simulink model "Date0501_QuadModel"  (R2015a)
settings: Solver=ode3  StartTime=0.0  StopTime=inf  FixedStep=Ts/5  RelTol=1e-3
values from neighbouring files (symbols this model uses):
  alpha1 = 10    [Date0501_Input_QuadModel.m]
  alpha2 = .3    (= 0.3)    [Date0501_Input_QuadModel.m]
  alpha3 = 1    [Date0501_Input_QuadModel.m]
  alpha4 = .1    (= 0.1)    [Date0501_Input_QuadModel.m]
  alpha5 = 1    [Date0501_Input_QuadModel.m]
  alpha6 = .1    (= 0.1)    [Date0501_Input_QuadModel.m]
  Am = - diag([10, 10, 10])*2    [Date0501_Input_QuadModel.m]
  Bm = diag([L_arm/Ix, L_arm/Iy, 1/Iz])    [Date0501_Input_QuadModel.m]
  Delay_Act = 0.0    (= 0)    [Date0501_Input_QuadModel.m]
  g = 9.81    [Date0501_Input_QuadModel.m]
  Inerita_Mat = diag([Ix, Iy, Iz])    [Date0501_Input_QuadModel.m]
  Ix = 7.5e-3    (= 0.0075)    [Date0501_Input_QuadModel.m]
  Iy = 7.5e-3    (= 0.0075)    [Date0501_Input_QuadModel.m]
  Jr = 6e-5    (= 6e-05)    [Date0501_Input_QuadModel.m]
  L_arm = 0.23    [Date0501_Input_QuadModel.m]
  m = 1.650    (= 1.65)    [Date0501_Input_QuadModel.m]
  Rotor_State_Fail = diag([1 1 1 0.5])    [Date0501_Input_QuadModel.m]
  Rotor_State_Normal = diag([1 1 1 1])    [Date0501_Input_QuadModel.m]
  Speed_Square_to_Thrust_N_Moment_Mat = [b b b b; 0 -b 0 b; -b 0 b 0; -d d -d d]    [Date0501_Input_QuadModel.m]
  Sum_Rotor_Angular_Velocity_Mat = [-1 1 -1 1]    [Date0501_Input_QuadModel.m]
  Ts = 0.005    [Date0501_Input_QuadModel.m]
libraries: simulink x8, cstblocks x4, etargetslib x1, aerolibutil x1, aerolibanimutils x1, dspnetwork x1
settings Model: SimulationMode=accelerator  Creator=hyoon33  LastModifiedBy=marinho
settings SolverCC: PositivePriorityOrder=on
settings DebuggingCC: UnderspecifiedInitializationDetection=Classic  MergeDetectMultiDrivingBlocksExec=none  SolverPrmCheckMsg=warning  StateNameClashWarn=warning

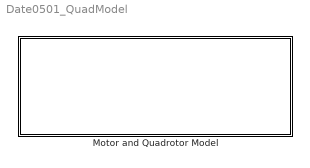
== system Date0501_QuadModel ==
  Motor and Quadrotor Model : Subsystem

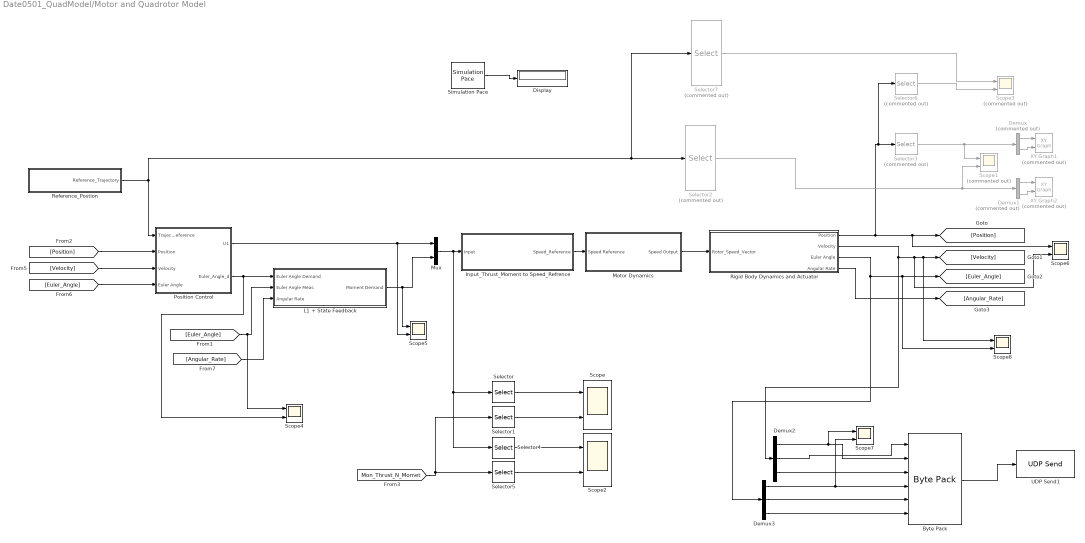
== system Date0501_QuadModel/Motor and Quadrotor Model ==
  Byte Pack : etargetslib/Byte Pack  datatypes={'double','double','double','double','double','double'}  byteAlign=1
  Demux : Demux  Commented=on  Outputs=2
  Demux1 : Demux  Commented=on  Outputs=2
  Demux2 : Demux  Outputs=3
  Demux3 : Demux  Outputs=3
  Display : Display
  Input_Thrust_Moment to Speed_Refrence : Subsystem
  L1 + State Feedback : Subsystem
  Motor Dynamics : Subsystem
  Mux : Mux  Inputs=2
  Position Control : Subsystem
  Reference_Postion : Subsystem
  Rigid Body Dynamics and Actuator : Subsystem
  Scope{,2,4..8} (7 alike) : Scope  NumInputPorts=2
      Scope settings: YMin=-0.6~-0.6  YMax=0.6~0.6
      Scope2 settings: YMin=6~6  YMax=13~13  SaveName=ScopeData11
      Scope4 settings: YMin=-0.175~-0.1  YMax=0.15~0.1  SaveName=ScopeData5
      Scope5 settings: YMin=-2.75~7.9  YMax=3~8.25  SaveName=ScopeData6
      Scope6 settings: YMin=-0.1~-0.7  YMax=1.3~0.6  SaveName=ScopeData7
      Scope7 settings: YMin=-1.5~-0.012  YMax=1.25~0.008  SaveName=ScopeData9
      Scope8 settings: YMin=-0.75~-0.075  YMax=1.25~0.125  SaveName=ScopeData10
  Scope1 : Scope  Commented=on  NumInputPorts=2
      settings: YMin=-0.8~-0.5  YMax=0.6~0.5  SaveName=ScopeData3
  Scope3 : Scope  Commented=on  NumInputPorts=2
      settings: YMin=1.02~0.91  YMax=1.095~0.985  SaveName=ScopeData12
  Selector : Selector  InputPortWidth=4  Indices=[2 3 4]
  Selector1 : Selector  InputPortWidth=4  Indices=[2 3 4]
  Selector2 : Selector  Commented=on  InputPortWidth=7  Indices=[3 5]
  Selector3 : Selector  Commented=on  InputPortWidth=3  Indices=[1 2]
  Selector4 : Selector  InputPortWidth=4  Indices=[1]
  Selector5 : Selector  InputPortWidth=4  Indices=[1]
  Selector6 : Selector  Commented=on  InputPortWidth=3  Indices=[3]
  Selector7 : Selector  Commented=on  InputPortWidth=7  Indices=[1]
  Simulation Pace : aerolibanimutils/Simulation Pace  SimulationPace=1  SleepMode=MATLAB Thread  OutputPaceError=on  SampleTime=-1
      settings: AttributesFormatString=%<SimulationPace> sec/sec
  UDP Send1 : dspnetwork/UDP Send  remoteURL='127.0.0.1'  remotePort=25000  localURL='0.0.0.0'  localPortSource=Automatically determine  localPort=-1  sampletime=-1  separateLengthPort=0
  XY Graph1 : simulink/Sinks/XY Graph  Commented=on  xmin=-2  xmax=2  ymin=-2  ymax=2  st=-1
  XY Graph2 : simulink/Sinks/XY Graph  Commented=on  xmin=-2  xmax=2  ymin=-2  ymax=2  st=-1
  wires:
  Rigid Body Dynamics and Actuator/4(Angular Rate) -> [Angular_Rate]
  Rigid Body Dynamics and Actuator/2(Velocity) -> Demux2/1, Scope6/2, Scope8/1, [Velocity]
  Rigid Body Dynamics and Actuator/1(Position) -> Selector6/1, Selector3/1, Scope6/1, [Position]
  Rigid Body Dynamics and Actuator/3(Euler Angle) -> Demux3/1, Scope8/2, [Euler_Angle]
  Input_Thrust_Moment to Speed_Refrence/1(Speed_Reference) -> Motor Dynamics/1(Speed Reference)
  L1 + State Feedback/1(Moment Demand) -> Scope5/1, Mux/2
  Reference_Postion/1(Reference_Trajectory) -> Position Control/1(Trajectory_Reference), Selector7/1, Selector2/1
  [Position] -> Position Control/2(Position)
  [Velocity] -> Position Control/3(Velocity)
  [Euler_Angle] -> Position Control/4(Euler Angle)
  [Euler_Angle] -> Scope4/1, L1 + State Feedback/2(Euler Angle Meas)
  [Angular_Rate] -> L1 + State Feedback/3(Angular Rate)
  Position Control/2(Euler_Angle_d) -> L1 + State Feedback/1(Euler Angle Demand), Scope4/2
  Mux/1 -> Selector/1, Selector4/1, Input_Thrust_Moment to Speed_Refrence/1(Input)
  Selector1/1 -> Scope/2
  Selector/1 -> Scope/1
  [Mon_Thrust_N_Momet] -> Selector5/1, Selector1/1
  Selector2/1 -> Scope1/2, Demux1/1
  Selector3/1 -> Scope1/1, Demux/1
  Selector4/1 -> Scope2/1
  Selector5/1 -> Scope2/2
  Selector6/1 -> Scope3/2
  Selector7/1 -> Scope3/1
  Position Control/1(U1) -> Mux/1, Scope5/2
  Demux1/1 -> XY Graph2/1
  Demux1/2 -> XY Graph2/2
  Demux/1 -> XY Graph1/1
  Demux/2 -> XY Graph1/2
  Byte Pack/1 -> UDP Send1/1
  Motor Dynamics/1(Speed Output) -> Rigid Body Dynamics and Actuator/1(Rotor_Speed_Vector)
  Simulation Pace/1 -> Display/1
  Demux2/1 -> Scope7/1, Byte Pack/2
  Demux3/2 -> Byte Pack/5
  Demux2/2 -> Byte Pack/1
  Demux3/1 -> Scope7/2, Byte Pack/4
  Demux2/3 -> Byte Pack/3
  Demux3/3 -> Byte Pack/6

== system Date0501_QuadModel/Motor and Quadrotor Model/Input_Thrust_Moment to Speed_Refrence ==
  Input : Inport
  From Speed 2 Thrust and Moment : Constant  Value=inv(Speed_Square_to_Thrust_N_Moment_Mat)  VectorParams1D=off
  Product : Product  Multiplication=Matrix(*)
  Speed_Reference : Outport
  wires:
  From Speed 2 Thrust and Moment/1 -> Product/1
  Product/1 -> Speed_Reference/1
  Input/1 -> Product/2

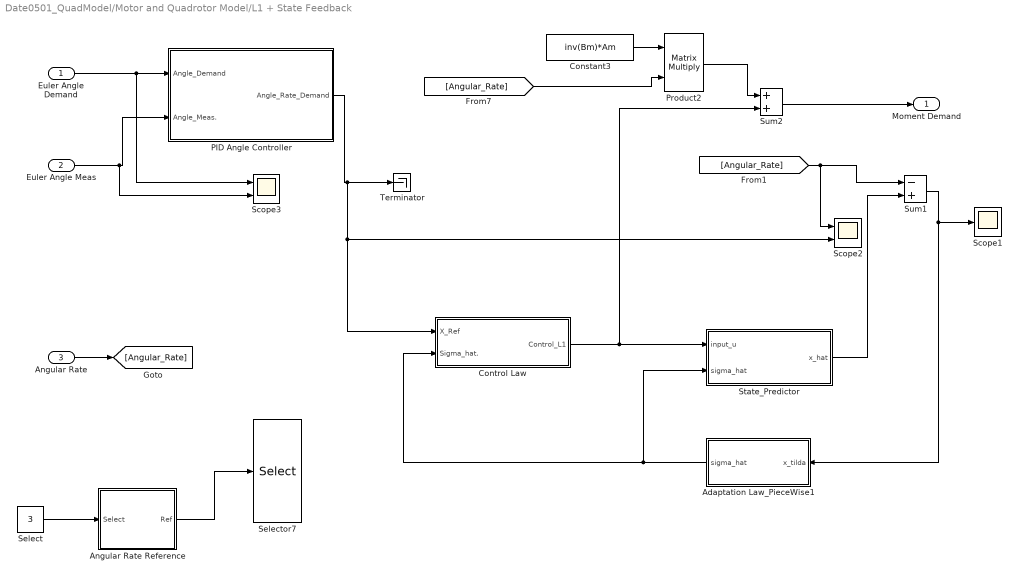
== system Date0501_QuadModel/Motor and Quadrotor Model/L1 + State Feedback ==
  Euler Angle Demand : Inport
  Euler Angle Meas : Inport  Port=2
  Angular Rate : Inport  Port=3
  Adaptation Law_PieceWise1 : Subsystem
  Angular Rate Reference : Subsystem
  Constant3 : Constant  Value=inv(Bm)*Am
  Control Law : Subsystem
  PID Angle Controller : Subsystem
  Product2 : Product  Multiplication=Matrix(*)
  Scope1 : Scope
      settings: YMin=-0.35  YMax=0.05  SaveName=ScopeData2
  Scope2 : Scope  NumInputPorts=2
      settings: YMin=-2~-3  YMax=2.5~3
  Scope3 : Scope  NumInputPorts=2
      settings: YMin=-1.75~-1.75  YMax=1.75~1.75  SaveName=ScopeData4
  Select : Constant  Value=3
  Selector7 : Selector  InputPortWidth=4  Indices=[1 2 3]
  State_Predictor : Subsystem
  Sum1 : Sum  Inputs=-+
  Sum2 : Sum
  Terminator : Terminator
  Moment Demand : Outport
  wires:
  Euler Angle Demand/1 -> Scope3/1, PID Angle Controller/1(Angle_Demand)
  Euler Angle Meas/1 -> Scope3/2, PID Angle Controller/2(Angle_Meas.)
  Angular Rate/1 -> [Angular_Rate]
  Sum1/1 -> Scope1/1, Adaptation Law_PieceWise1/1(x_tilda)
  State_Predictor/1(x_hat) -> Sum1/2
  Adaptation Law_PieceWise1/1(sigma_hat) -> State_Predictor/2(sigma_hat), Control Law/2(Sigma_hat.)
  PID Angle Controller/1(Angle_Rate_Demand) -> Scope2/2, Control Law/1(X_Ref), Terminator/1
  Constant3/1 -> Product2/1
  [Angular_Rate] -> Product2/2
  Sum2/1 -> Moment Demand/1
  Product2/1 -> Sum2/1
  Control Law/1(Control_L1) -> Sum2/2, State_Predictor/1(input_u)
  [Angular_Rate] -> Scope2/1, Sum1/1
  Select/1 -> Angular Rate Reference/1(Select)
  Angular Rate Reference/1(Ref) -> Selector7/1

== system Date0501_QuadModel/Motor and Quadrotor Model/Motor Dynamics ==
  Speed Reference : Inport
  Demux : Demux
  LTI System{1..4} (4 alike) : cstblocks/LTI System  sys=G_motor  IC=[]
  Mux : Mux
  Transport Delay : TransportDelay  DelayTime=Delay_Act
  Speed Output : Outport
  wires:
  Speed Reference/1 -> Transport Delay/1
  Transport Delay/1 -> Demux/1
  Mux/1 -> Speed Output/1
  Demux/1 -> LTI System1/1
  LTI System1/1 -> Mux/1
  Demux/2 -> LTI System2/1
  LTI System2/1 -> Mux/2
  Demux/3 -> LTI System3/1
  LTI System3/1 -> Mux/3
  Demux/4 -> LTI System4/1
  LTI System4/1 -> Mux/4

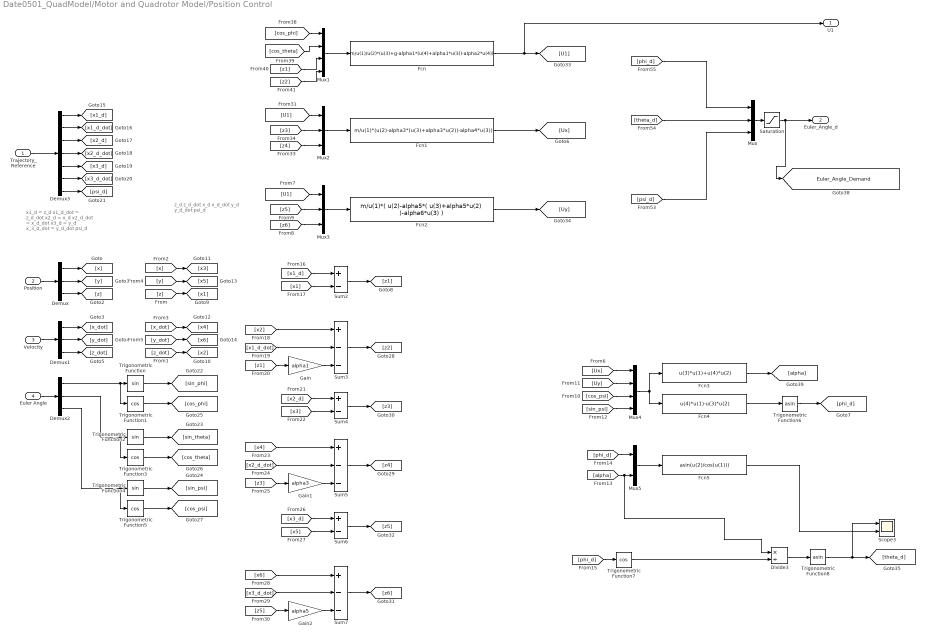
== system Date0501_QuadModel/Motor and Quadrotor Model/Position Control ==
  note: x1_d =  z_d
      | x1_d_dot = z_d_dot
      |
      | x2_d = x_d
      | x2_d_dot = x_d_dot
      |
      | x3_d = y_d
      | x_3_d_dot = y_d_dot
      |
      | psi_d
  note: z_d
      | z_d_dot
      |
      | x_d
      | x_d_dot
      |
      | y_d
      | y_d_dot
      |
      | psi_d
  Trajectory_Reference : Inport
  Position : Inport  Port=2
  Velocity : Inport  Port=3
  Euler Angle : Inport  Port=4
  Demux : Demux  Outputs=3
  Demux1 : Demux  Outputs=3
  Demux2 : Demux  Outputs=3
  Demux3 : Demux  Outputs=7
  Divide3 : Product  Inputs=*/
  Fcn : Fcn  Expr=m/u(1)/u(2)*(u(3)+g-alpha1*(u(4)+alpha1*u(3))-alpha2*u(4))
  Fcn1 : Fcn  Expr=m/u(1)*(u(2)-alpha3*(u(3)+alpha3*u(2))-alpha4*u(3))
  Fcn2 : Fcn  Expr=m/u(1)*( u(2)-alpha5*( u(3)+alpha5*u(2) )-alpha6*u(3) )
  Fcn3 : Fcn  Expr=u(3)*u(1)+u(4)*u(2)
  Fcn4 : Fcn  Expr=u(4)*u(1)-u(3)*u(2)
  Fcn5 : Fcn  Expr=asin(u(2)/cos(u(1)))
  Gain : Gain  Gain=alpha1
  Gain1 : Gain  Gain=alpha3
  Gain2 : Gain  Gain=alpha5
  Mux : Mux  Inputs=3
  Mux1 : Mux
  Mux2 : Mux  Inputs=3
  Mux3 : Mux  Inputs=3
  Mux4 : Mux
  Mux5 : Mux  Inputs=2
  Saturation : Saturate  UpperLimit=0.1  LowerLimit=-0.1
  Scope3 : Scope  NumInputPorts=2
      settings: YMin=-5~-5  YMax=5~5  SaveName=ScopeData8
  Sum2 : Sum  Inputs=+-
  Sum3 : Sum  Inputs=+--
  Sum4 : Sum  Inputs=+-
  Sum5 : Sum  Inputs=+--
  Sum6 : Sum  Inputs=+-
  Sum7 : Sum  Inputs=+--
  Trigonometric Function : Trigonometry
  Trigonometric Function{1,3,5,7} (4 alike) : Trigonometry  Operator=cos
  Trigonometric Function2 : Trigonometry
  Trigonometric Function4 : Trigonometry
  Trigonometric Function6 : Trigonometry  Operator=asin
  Trigonometric Function8 : Trigonometry  Operator=asin
  U1 : Outport
  Euler_Angle_d : Outport  Port=2
  tag scope: Euler_Angle_Demand=global
  wires:
  Position/1 -> Demux/1
  Velocity/1 -> Demux1/1
  Euler Angle/1 -> Demux2/1
  Demux/1 -> [x]
  Demux/2 -> [y]
  Demux/3 -> [z]
  Demux1/1 -> [x_dot]
  Demux1/2 -> [y_dot]
  Demux1/3 -> [z_dot]
  [z] -> [x1]
  [z_dot] -> [x2]
  [x] -> [x3]
  [x_dot] -> [x4]
  [y] -> [x5]
  [y_dot] -> [x6]
  Trajectory_Reference/1 -> Demux3/1
  Demux3/1 -> [x1_d]
  Demux3/2 -> [x1_d_dot]
  Demux3/3 -> [x2_d]
  Demux3/4 -> [x2_d_dot]
  Demux3/5 -> [x3_d]
  Demux3/6 -> [x3_d_dot]
  Demux3/7 -> [psi_d]
  Demux2/1 -> Trigonometric Function1/1, Trigonometric Function/1
  Trigonometric Function/1 -> [sin_phi]
  Trigonometric Function1/1 -> [cos_phi]
  Demux2/2 -> Trigonometric Function3/1, Trigonometric Function2/1
  Trigonometric Function2/1 -> [sin_theta]
  Trigonometric Function3/1 -> [cos_theta]
  Trigonometric Function4/1 -> [sin_psi]
  Trigonometric Function5/1 -> [cos_psi]
  Demux2/3 -> Trigonometric Function5/1, Trigonometric Function4/1
  [x1_d] -> Sum2/1
  [x1] -> Sum2/2
  Sum2/1 -> [z1]
  [x1_d_dot] -> Sum3/2
  [x2] -> Sum3/1
  Gain/1 -> Sum3/3
  [z1] -> Gain/1
  Sum3/1 -> [z2]
  [x2_d] -> Sum4/1
  [x3] -> Sum4/2
  Sum4/1 -> [z3]
  [x2_d_dot] -> Sum5/2
  [x4] -> Sum5/1
  Gain1/1 -> Sum5/3
  [z3] -> Gain1/1
  Sum5/1 -> [z4]
  [x3_d] -> Sum6/1
  [x5] -> Sum6/2
  Sum6/1 -> [z5]
  [x3_d_dot] -> Sum7/2
  [x6] -> Sum7/1
  Gain2/1 -> Sum7/3
  [z5] -> Gain2/1
  Sum7/1 -> [z6]
  Mux/1 -> Saturation/1
  [alpha] -> Divide3/1, Mux5/2
  Trigonometric Function7/1 -> Divide3/2
  Divide3/1 -> Trigonometric Function8/1
  Trigonometric Function8/1 -> Scope3/1, [theta_d]
  Mux1/1 -> Fcn/1
  [cos_phi] -> Mux1/1
  [cos_theta] -> Mux1/2
  [z1] -> Mux1/3
  [z2] -> Mux1/4
  Mux2/1 -> Fcn1/1
  [U1] -> Mux2/1
  [z4] -> Mux2/3
  [z3] -> Mux2/2
  Fcn1/1 -> [Ux]
  Mux3/1 -> Fcn2/1
  [U1] -> Mux3/1
  [z6] -> Mux3/3
  [z5] -> Mux3/2
  Fcn2/1 -> [Uy]
  Mux4/1 -> Fcn4/1, Fcn3/1
  [Ux] -> Mux4/1
  [cos_psi] -> Mux4/3
  [Uy] -> Mux4/2
  [sin_psi] -> Mux4/4
  Fcn4/1 -> Trigonometric Function6/1
  Trigonometric Function6/1 -> [phi_d]
  Fcn3/1 -> [alpha]
  [phi_d] -> Mux5/1
  Mux5/1 -> Fcn5/1
  Fcn5/1 -> Scope3/2
  [phi_d] -> Trigonometric Function7/1
  [phi_d] -> Mux/1
  [theta_d] -> Mux/2
  [psi_d] -> Mux/3
  Fcn/1 -> U1/1, [U1]
  Saturation/1 -> [Euler_Angle_Demand], Euler_Angle_d/1

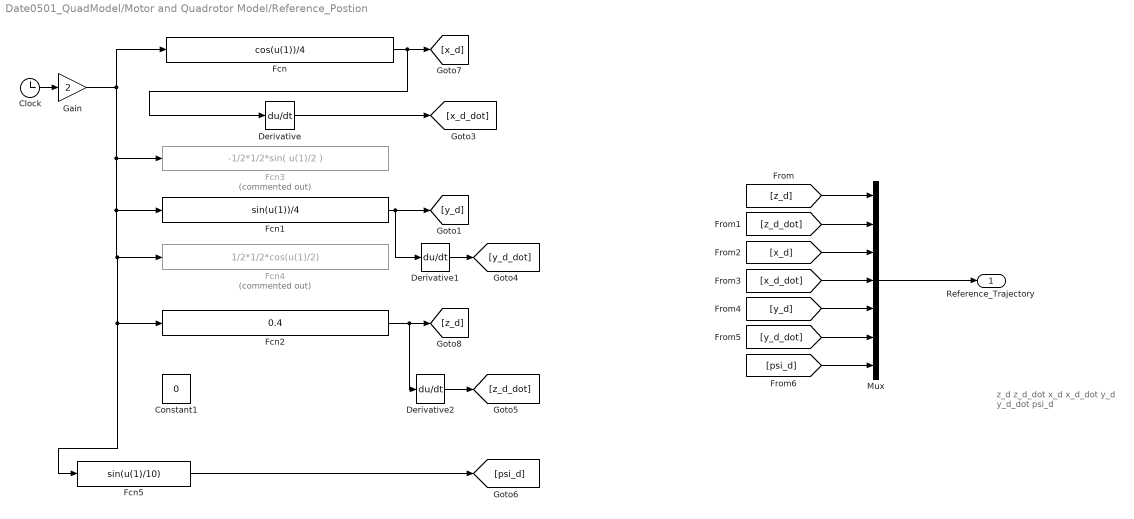
== system Date0501_QuadModel/Motor and Quadrotor Model/Reference_Postion ==
  note: z_d
      | z_d_dot
      |
      | x_d
      | x_d_dot
      |
      | y_d
      | y_d_dot
      |
      | psi_d
  Clock : Clock
  Constant1 : Constant  Value=0
  Derivative : Derivative
  Derivative1 : Derivative
  Derivative2 : Derivative
  Fcn : Fcn  Expr=cos(u(1))/4
  Fcn1 : Fcn  Expr=sin(u(1))/4
  Fcn2 : Fcn  Expr=0.4
  Fcn3 : Fcn  Commented=on  Expr=-1/2*1/2*sin( u(1)/2 )
  Fcn4 : Fcn  Commented=on  Expr=1/2*1/2*cos(u(1)/2)
  Fcn5 : Fcn  Expr=sin(u(1)/10)
  Gain : Gain  Gain=2
  Mux : Mux  Inputs=7
  Reference_Trajectory : Outport
  wires:
  Clock/1 -> Gain/1
  Fcn5/1 -> [psi_d]
  Mux/1 -> Reference_Trajectory/1
  [z_d] -> Mux/1
  [z_d_dot] -> Mux/2
  [x_d] -> Mux/3
  [x_d_dot] -> Mux/4
  [y_d] -> Mux/5
  [y_d_dot] -> Mux/6
  [psi_d] -> Mux/7
  Fcn2/1 -> Derivative2/1, [z_d]
  Gain/1 -> Fcn1/1, Fcn4/1, Fcn5/1, Fcn2/1, Fcn3/1, Fcn/1
  Fcn/1 -> [x_d], Derivative/1
  Derivative2/1 -> [z_d_dot]
  Fcn1/1 -> [y_d], Derivative1/1
  Derivative1/1 -> [y_d_dot]
  Derivative/1 -> [x_d_dot]

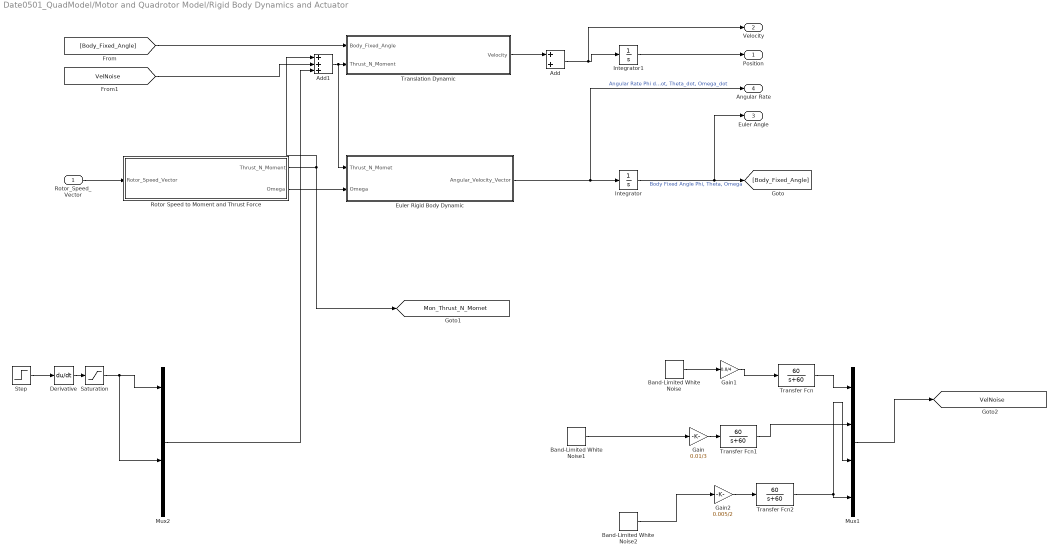
== system Date0501_QuadModel/Motor and Quadrotor Model/Rigid Body Dynamics and Actuator ==
  Rotor_Speed_Vector : Inport
  Add : Sum
  Add1 : Sum  Inputs=+++
  Band-Limited White Noise : simulink/Sources/Band-Limited White Noise  Cov=[.1]  Ts=Ts/5  seed=[23341]
  Band-Limited White Noise1 : simulink/Sources/Band-Limited White Noise  Cov=[.1]  Ts=Ts/5  seed=[24451]
  Band-Limited White Noise2 : simulink/Sources/Band-Limited White Noise  Cov=[.1]  Ts=Ts/5  seed=[87745]
  Derivative : Derivative
  Euler Rigid Body Dynamic : Subsystem
  Gain : Gain  Gain=0.01/3
  Gain1 : Gain  Gain=0.8/4
  Gain2 : Gain  Gain=0.005/2
  Integrator : Integrator
  Integrator1 : Integrator  InitialCondition=[0, 0, 0.5]'
  Mux1 : Mux
  Mux2 : Mux
  Rotor Speed to Moment and Thrust Force : Subsystem
  Saturation : Saturate  UpperLimit=10  LowerLimit=-10
  Step : Step  Time=20  SampleTime=0
  Transfer Fcn : TransferFcn  Numerator=[60]  Denominator=[1 60]
  Transfer Fcn1 : TransferFcn  Numerator=[60]  Denominator=[1 60]
  Transfer Fcn2 : TransferFcn  Numerator=[60]  Denominator=[1 60]
  Translation Dynamic : Subsystem
  Position : Outport
  Velocity : Outport  Port=2
  Euler Angle : Outport  Port=3
  Angular Rate : Outport  Port=4
  tag scope: Mon_Thrust_N_Momet=global, VelNoise=global
  wires:
  Rotor Speed to Moment and Thrust Force/1(Thrust_N_Moment) -> Add1/1, [Mon_Thrust_N_Momet]
  Euler Rigid Body Dynamic/1(Angular_Velocity_Vector) -> Integrator/1, Angular Rate/1  "Angular Rate Phi dot, Theta_dot, Omega_dot"
  Integrator/1 -> Euler Angle/1, [Body_Fixed_Angle]  "Body Fixed Angle Phi, Theta, Omega"
  Integrator1/1 -> Position/1
  Rotor Speed to Moment and Thrust Force/2(Omega) -> Euler Rigid Body Dynamic/2(Omega)
  Rotor_Speed_Vector/1 -> Rotor Speed to Moment and Thrust Force/1(Rotor_Speed_Vector)
  [Body_Fixed_Angle] -> Translation Dynamic/1(Body_Fixed_Angle)
  Band-Limited White Noise/1 -> Gain1/1
  Band-Limited White Noise1/1 -> Gain/1
  Band-Limited White Noise2/1 -> Gain2/1
  Mux1/1 -> [VelNoise]
  Gain/1 -> Transfer Fcn1/1
  Gain1/1 -> Transfer Fcn/1
  Gain2/1 -> Transfer Fcn2/1
  Translation Dynamic/1(Velocity) -> Add/1
  Add/1 -> Velocity/1, Integrator1/1
  Add1/1 -> Euler Rigid Body Dynamic/1(Thrust_N_Momet), Translation Dynamic/2(Thrust_N_Moment)
  Transfer Fcn/1 -> Mux1/1
  Transfer Fcn1/1 -> Mux1/2
  Transfer Fcn2/1 -> Mux1/3, Mux1/4
  [VelNoise] -> Add1/2
  Mux2/1 -> Add1/3
  Step/1 -> Derivative/1
  Derivative/1 -> Saturation/1
  Saturation/1 -> Mux2/3, Mux2/1

== system Date0501_QuadModel/Motor and Quadrotor Model/L1 + State Feedback/Adaptation Law_PieceWise1 ==
  x_tilda : Inport
  -inv(Bm)*inv(Phi_Ts)*exp_Am_Ts : Constant  Value=inv(Bm)*inv(inv(Am)*(expm(Am*Ts)-eye(3)))*(expm(Am*Ts))
  Gain3 : Gain  Gain=-1
  Product6 : Product  Multiplication=Matrix(*)
  Rate Transition : RateTransition  OutPortSampleTime=Ts
  Rate Transition1 : RateTransition  OutPortSampleTimeOpt=Inherit  OutPortSampleTime=Ts
  Rate Transition3 : RateTransition  X0=inv(Bm)*inv(inv(Am)*(exp(Am*Ts)-eye(3)))*(exp(Am*Ts))  OutPortSampleTime=Ts
  Saturation2 : Saturate  UpperLimit=10000  LowerLimit=-10000
  sigma_hat : Outport
  wires:
  Saturation2/1 -> sigma_hat/1
  Rate Transition3/1 -> Product6/1
  Gain3/1 -> Rate Transition1/1
  Rate Transition1/1 -> Saturation2/1
  -inv(Bm)*inv(Phi_Ts)*exp_Am_Ts/1 -> Rate Transition3/1
  x_tilda/1 -> Rate Transition/1
  Product6/1 -> Gain3/1
  Rate Transition/1 -> Product6/2

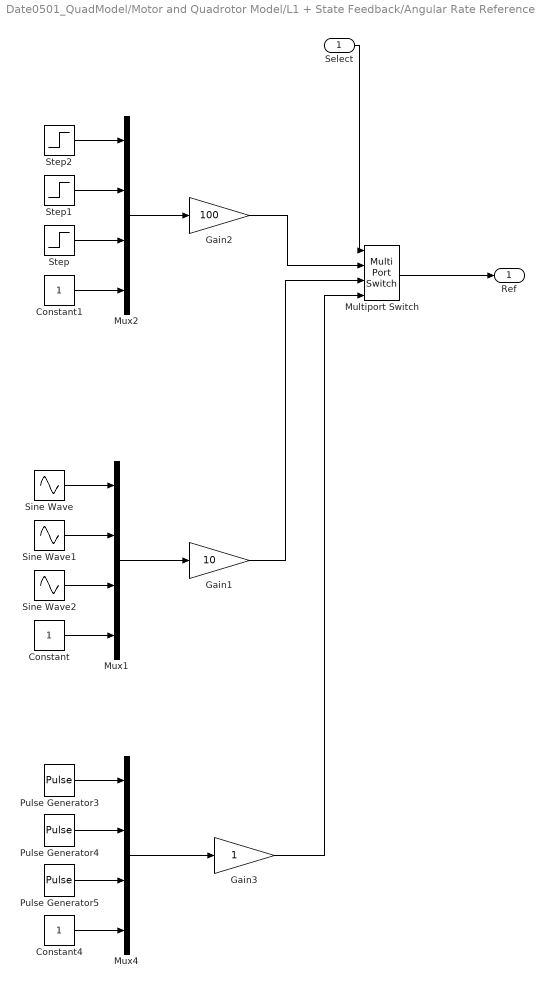
== system Date0501_QuadModel/Motor and Quadrotor Model/L1 + State Feedback/Angular Rate Reference ==
  Select : Inport
  Constant : Constant
  Constant1 : Constant
  Constant4 : Constant
  Gain1 : Gain  Gain=10
  Gain2 : Gain  Gain=100
  Gain3 : Gain
  Multiport Switch : MultiPortSwitch
  Mux1 : Mux
  Mux2 : Mux
  Mux4 : Mux
  Pulse Generator3 : DiscretePulseGenerator  PulseType=Time based  Period=8  PulseWidth=40  PhaseDelay=1
  Pulse Generator4 : DiscretePulseGenerator  PulseType=Time based  Period=8  PulseWidth=40  PhaseDelay=1.5
  Pulse Generator5 : DiscretePulseGenerator  PulseType=Time based  Amplitude=0  Period=8  PulseWidth=40  PhaseDelay=2
  Sine Wave : Sin  SampleTime=0
  Sine Wave1 : Sin  Phase=pi  SampleTime=0
  Sine Wave2 : Sin  Amplitude=0  SampleTime=0
  Step : Step  Time=3  After=0  SampleTime=0
  Step1 : Step  Time=2  SampleTime=0
  Step2 : Step  SampleTime=0
  Ref : Outport
  wires:
  Sine Wave/1 -> Mux1/1
  Sine Wave1/1 -> Mux1/2
  Sine Wave2/1 -> Mux1/3
  Constant/1 -> Mux1/4
  Step2/1 -> Mux2/1
  Step1/1 -> Mux2/2
  Step/1 -> Mux2/3
  Constant1/1 -> Mux2/4
  Mux1/1 -> Gain1/1
  Mux2/1 -> Gain2/1
  Select/1 -> Multiport Switch/1
  Gain2/1 -> Multiport Switch/2
  Multiport Switch/1 -> Ref/1
  Pulse Generator3/1 -> Mux4/1
  Pulse Generator4/1 -> Mux4/2
  Pulse Generator5/1 -> Mux4/3
  Constant4/1 -> Mux4/4
  Mux4/1 -> Gain3/1
  Gain1/1 -> Multiport Switch/3
  Gain3/1 -> Multiport Switch/4

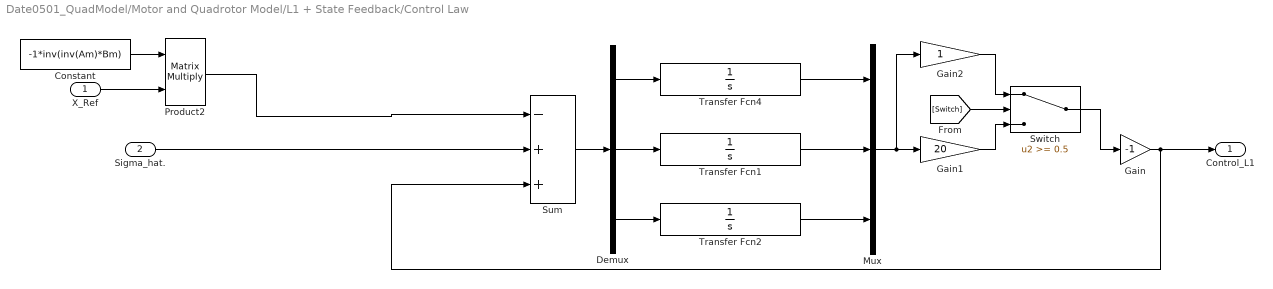
== system Date0501_QuadModel/Motor and Quadrotor Model/L1 + State Feedback/Control Law ==
  X_Ref : Inport
  Sigma_hat. : Inport  Port=2
  Constant : Constant  Value=-1*inv(inv(Am)*Bm)
  Demux : Demux  Outputs=3
  Gain : Gain  Gain=-1
  Gain1 : Gain  Gain=20
  Gain2 : Gain
  Mux : Mux  Inputs=3
  Product2 : Product  Multiplication=Matrix(*)
  Sum : Sum  Inputs=-++
  Switch : Switch  Threshold=0.5
  Transfer Fcn1 : TransferFcn  Denominator=[1 0]
  Transfer Fcn2 : TransferFcn  Denominator=[1 0]
  Transfer Fcn4 : TransferFcn  Denominator=[1 0]
  Control_L1 : Outport
  wires:
  X_Ref/1 -> Product2/2
  Sum/1 -> Demux/1
  Demux/1 -> Transfer Fcn4/1
  Demux/2 -> Transfer Fcn1/1
  Demux/3 -> Transfer Fcn2/1
  Mux/1 -> Gain2/1, Gain1/1
  Transfer Fcn4/1 -> Mux/1
  Transfer Fcn1/1 -> Mux/2
  Transfer Fcn2/1 -> Mux/3
  Constant/1 -> Product2/1
  Gain1/1 -> Switch/3
  Sigma_hat./1 -> Sum/2
  Gain/1 -> Sum/3, Control_L1/1
  Product2/1 -> Sum/1
  Gain2/1 -> Switch/1
  Switch/1 -> Gain/1
  [Switch] -> Switch/2

== system Date0501_QuadModel/Motor and Quadrotor Model/L1 + State Feedback/PID Angle Controller ==
  Angle_Demand : Inport
  Angle_Meas. : Inport  Port=2
  Demux : Demux  Outputs=3
  Demux1 : Demux  Outputs=3
  Mux : Mux  Inputs=3
  PID Controller (2DOF) : simulink/Continuous/PID Controller (2DOF)  Controller=PID  TimeDomain=Continuous-time  SampleTime=-1  IntegratorMethod=Forward Euler  FilterMethod=Forward Euler  Form=Parallel  UseFilter=on  ControllerParametersSource=internal  P=10  I=0.1  D=0.01  N=100  b=1  c=1  InitialConditionSource=internal  InitialConditionForIntegrator=0  InitialConditionForFilter=0  ExternalReset=none  LimitOutput=off  UpperSaturationLimit=inf  LowerSaturationLimit=-inf  LinearizeAsGain=on  AntiWindupMode=none  Kb=1  TrackingMode=off  Kt=1  PParamMin=[]  PParamMax=[]  IParamMin=[]  IParamMax=[]  DParamMin=[]  DParamMax=[]  NParamMin=[]  NParamMax=[]  bParamMin=[]  bParamMax=[]  cParamMin=[]  cParamMax=[]  KbParamMin=[]  KbParamMax=[]  KtParamMin=[]  KtParamMax=[]  POutMin=[]  POutMax=[]  IOutMin=[]  IOutMax=[]  DOutMin=[]  DOutMax=[]  NOutMin=[]  NOutMax=[]  bOutMin=[]  bOutMax=[]  cOutMin=[]  cOutMax=[]  KbOutMin=[]  KbOutMax=[]  KtOutMin=[]  KtOutMax=[]  IntegratorOutMin=[]  IntegratorOutMax=[]  FilterOutMin=[]  FilterOutMax=[]  SumOutMin=[]  SumOutMax=[]  Sum1OutMin=[]  Sum1OutMax=[]  Sum2OutMin=[]  Sum2OutMax=[]  Sum3OutMin=[]  Sum3OutMax=[]  SumI1OutMin=[]  SumI1OutMax=[]  SumI2OutMin=[]  SumI2OutMax=[]  SumI3OutMin=[]  SumI3OutMax=[]  SumDOutMin=[]  SumDOutMax=[]  SaturationOutMin=[]  SaturationOutMax=[]  IntegratorContinuousStateAttributes=''  IntegratorStateMustResolveToSignalObject=off  IntegratorRTWStateStorageClass=Auto  FilterContinuousStateAttributes=''  FilterStateMustResolveToSignalObject=off  FilterRTWStateStorageClass=Auto  DifferentiatorICPrevScaledInput=0  DifferentiatorOutMin=[]  DifferentiatorOutMax=[]
  PID Controller (2DOF)1 : simulink/Continuous/PID Controller (2DOF)  Controller=PID  TimeDomain=Continuous-time  SampleTime=-1  IntegratorMethod=Forward Euler  FilterMethod=Forward Euler  Form=Parallel  UseFilter=on  ControllerParametersSource=internal  P=10  I=0.1  D=0.01  N=100  b=1  c=1  InitialConditionSource=internal  InitialConditionForIntegrator=0  InitialConditionForFilter=0  ExternalReset=none  LimitOutput=off  UpperSaturationLimit=inf  LowerSaturationLimit=-inf  LinearizeAsGain=on  AntiWindupMode=none  Kb=1  TrackingMode=off  Kt=1  PParamMin=[]  PParamMax=[]  IParamMin=[]  IParamMax=[]  DParamMin=[]  DParamMax=[]  NParamMin=[]  NParamMax=[]  bParamMin=[]  bParamMax=[]  cParamMin=[]  cParamMax=[]  KbParamMin=[]  KbParamMax=[]  KtParamMin=[]  KtParamMax=[]  POutMin=[]  POutMax=[]  IOutMin=[]  IOutMax=[]  DOutMin=[]  DOutMax=[]  NOutMin=[]  NOutMax=[]  bOutMin=[]  bOutMax=[]  cOutMin=[]  cOutMax=[]  KbOutMin=[]  KbOutMax=[]  KtOutMin=[]  KtOutMax=[]  IntegratorOutMin=[]  IntegratorOutMax=[]  FilterOutMin=[]  FilterOutMax=[]  SumOutMin=[]  SumOutMax=[]  Sum1OutMin=[]  Sum1OutMax=[]  Sum2OutMin=[]  Sum2OutMax=[]  Sum3OutMin=[]  Sum3OutMax=[]  SumI1OutMin=[]  SumI1OutMax=[]  SumI2OutMin=[]  SumI2OutMax=[]  SumI3OutMin=[]  SumI3OutMax=[]  SumDOutMin=[]  SumDOutMax=[]  SaturationOutMin=[]  SaturationOutMax=[]  IntegratorContinuousStateAttributes=''  IntegratorStateMustResolveToSignalObject=off  IntegratorRTWStateStorageClass=Auto  FilterContinuousStateAttributes=''  FilterStateMustResolveToSignalObject=off  FilterRTWStateStorageClass=Auto  DifferentiatorICPrevScaledInput=0  DifferentiatorOutMin=[]  DifferentiatorOutMax=[]
  PID Controller (2DOF)2 : simulink/Continuous/PID Controller (2DOF)  Controller=PID  TimeDomain=Continuous-time  SampleTime=-1  IntegratorMethod=Forward Euler  FilterMethod=Forward Euler  Form=Parallel  UseFilter=on  ControllerParametersSource=internal  P=1  I=0.1  D=0.01  N=100  b=1  c=1  InitialConditionSource=internal  InitialConditionForIntegrator=0  InitialConditionForFilter=0  ExternalReset=none  LimitOutput=off  UpperSaturationLimit=inf  LowerSaturationLimit=-inf  LinearizeAsGain=on  AntiWindupMode=none  Kb=1  TrackingMode=off  Kt=1  PParamMin=[]  PParamMax=[]  IParamMin=[]  IParamMax=[]  DParamMin=[]  DParamMax=[]  NParamMin=[]  NParamMax=[]  bParamMin=[]  bParamMax=[]  cParamMin=[]  cParamMax=[]  KbParamMin=[]  KbParamMax=[]  KtParamMin=[]  KtParamMax=[]  POutMin=[]  POutMax=[]  IOutMin=[]  IOutMax=[]  DOutMin=[]  DOutMax=[]  NOutMin=[]  NOutMax=[]  bOutMin=[]  bOutMax=[]  cOutMin=[]  cOutMax=[]  KbOutMin=[]  KbOutMax=[]  KtOutMin=[]  KtOutMax=[]  IntegratorOutMin=[]  IntegratorOutMax=[]  FilterOutMin=[]  FilterOutMax=[]  SumOutMin=[]  SumOutMax=[]  Sum1OutMin=[]  Sum1OutMax=[]  Sum2OutMin=[]  Sum2OutMax=[]  Sum3OutMin=[]  Sum3OutMax=[]  SumI1OutMin=[]  SumI1OutMax=[]  SumI2OutMin=[]  SumI2OutMax=[]  SumI3OutMin=[]  SumI3OutMax=[]  SumDOutMin=[]  SumDOutMax=[]  SaturationOutMin=[]  SaturationOutMax=[]  IntegratorContinuousStateAttributes=''  IntegratorStateMustResolveToSignalObject=off  IntegratorRTWStateStorageClass=Auto  FilterContinuousStateAttributes=''  FilterStateMustResolveToSignalObject=off  FilterRTWStateStorageClass=Auto  DifferentiatorICPrevScaledInput=0  DifferentiatorOutMin=[]  DifferentiatorOutMax=[]
  Angle_Rate_Demand : Outport
  wires:
  Demux1/2 -> PID Controller (2DOF)1/2
  Demux/2 -> PID Controller (2DOF)1/1
  Angle_Meas./1 -> Demux1/1
  Demux1/1 -> PID Controller (2DOF)/2
  Demux/1 -> PID Controller (2DOF)/1
  Demux1/3 -> PID Controller (2DOF)2/2
  Angle_Demand/1 -> Demux/1
  Demux/3 -> PID Controller (2DOF)2/1
  PID Controller (2DOF)/1 -> Mux/1
  PID Controller (2DOF)1/1 -> Mux/2
  PID Controller (2DOF)2/1 -> Mux/3
  Mux/1 -> Angle_Rate_Demand/1

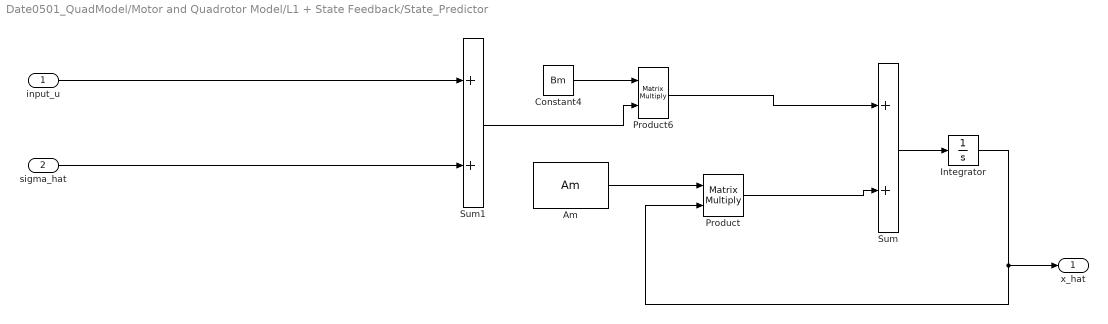
== system Date0501_QuadModel/Motor and Quadrotor Model/L1 + State Feedback/State_Predictor ==
  input_u : Inport
  sigma_hat : Inport  Port=2
  Am : Constant  Value=Am
  Constant4 : Constant  Value=Bm
  Integrator : Integrator
  Product : Product  Multiplication=Matrix(*)  RndMeth=Zero
  Product6 : Product  Multiplication=Matrix(*)
  Sum : Sum
  Sum1 : Sum
  x_hat : Outport
  wires:
  Product6/1 -> Sum/1
  Product/1 -> Sum/2
  Sum1/1 -> Product6/2
  Constant4/1 -> Product6/1
  Sum/1 -> Integrator/1
  input_u/1 -> Sum1/1
  Am/1 -> Product/1
  Integrator/1 -> x_hat/1, Product/2
  sigma_hat/1 -> Sum1/2

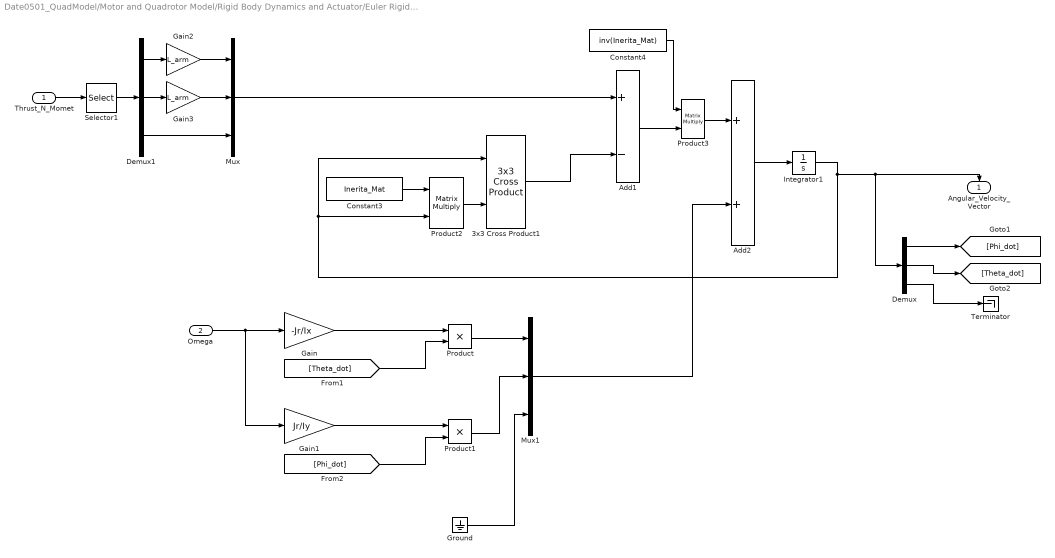
== system Date0501_QuadModel/Motor and Quadrotor Model/Rigid Body Dynamics and Actuator/Euler Rigid Body Dynamic ==
  Thrust_N_Momet : Inport
  Omega : Inport  Port=2
  3x3 Cross Product1 : aerolibutil/3x3 Cross Product
  Add1 : Sum  Inputs=+-
  Add2 : Sum
  Constant3 : Constant  Value=Inerita_Mat
  Constant4 : Constant  Value=inv(Inerita_Mat)
  Demux : Demux  Outputs=3
  Demux1 : Demux  Outputs=3
  Gain : Gain  Gain=-Jr/Ix
  Gain1 : Gain  Gain=Jr/Iy
  Gain2 : Gain  Gain=L_arm
  Gain3 : Gain  Gain=L_arm
  Ground : Ground
  Integrator1 : Integrator  InitialCondition=[0 0 0]
  Mux : Mux  Inputs=3
  Mux1 : Mux  Inputs=3
  Product : Product
  Product1 : Product
  Product2 : Product  Multiplication=Matrix(*)
  Product3 : Product  Multiplication=Matrix(*)
  Selector1 : Selector  InputPortWidth=4  Indices=[2 3 4]
  Terminator : Terminator
  Angular_Velocity_Vector : Outport
  wires:
  Add1/1 -> Product3/2
  3x3 Cross Product1/1 -> Add1/2
  Constant3/1 -> Product2/1
  Product2/1 -> 3x3 Cross Product1/2
  Constant4/1 -> Product3/1
  Thrust_N_Momet/1 -> Selector1/1
  Integrator1/1 -> Angular_Velocity_Vector/1, Demux/1, 3x3 Cross Product1/1, Product2/2
  Demux/1 -> [Phi_dot]
  Demux/2 -> [Theta_dot]
  Demux/3 -> Terminator/1
  Gain/1 -> Product/1
  Omega/1 -> Gain1/1, Gain/1
  [Theta_dot] -> Product/2
  Gain1/1 -> Product1/1
  [Phi_dot] -> Product1/2
  Selector1/1 -> Demux1/1
  Gain2/1 -> Mux/1
  Demux1/1 -> Gain2/1
  Demux1/2 -> Gain3/1
  Gain3/1 -> Mux/2
  Demux1/3 -> Mux/3
  Mux/1 -> Add1/1
  Product/1 -> Mux1/1
  Product1/1 -> Mux1/2
  Ground/1 -> Mux1/3
  Product3/1 -> Add2/1
  Add2/1 -> Integrator1/1
  Mux1/1 -> Add2/2

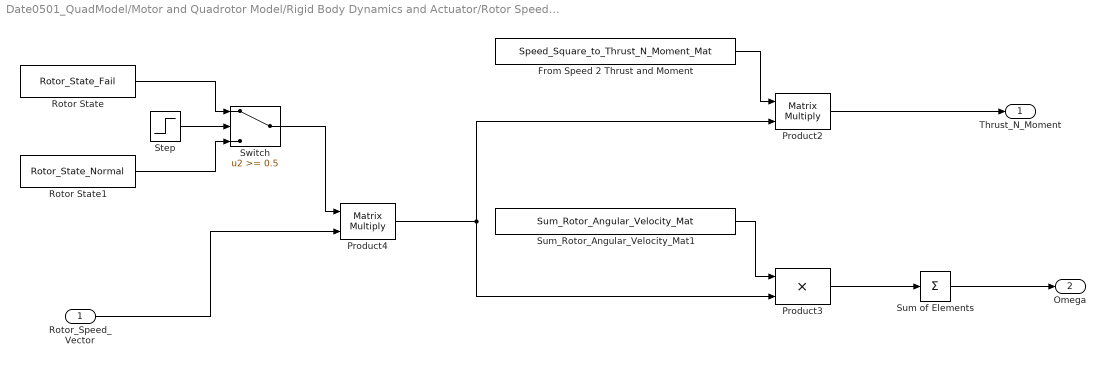
== system Date0501_QuadModel/Motor and Quadrotor Model/Rigid Body Dynamics and Actuator/Rotor Speed to Moment and Thrust Force ==
  Rotor_Speed_Vector : Inport
  From Speed 2 Thrust and Moment : Constant  Value=Speed_Square_to_Thrust_N_Moment_Mat
  Product2 : Product  Multiplication=Matrix(*)
  Product3 : Product
  Product4 : Product  Multiplication=Matrix(*)
  Rotor State : Constant  Value=Rotor_State_Fail
  Rotor State1 : Constant  Value=Rotor_State_Normal
  Step : Step  Time=10  SampleTime=0
  Sum of Elements : Sum  Inputs=+
  Sum_Rotor_Angular_Velocity_Mat1 : Constant  Value=Sum_Rotor_Angular_Velocity_Mat
  Switch : Switch  Threshold=0.5
  Thrust_N_Moment : Outport
  Omega : Outport  Port=2
  wires:
  From Speed 2 Thrust and Moment/1 -> Product2/1
  Rotor State/1 -> Switch/1
  Product4/1 -> Product2/2, Product3/2
  Switch/1 -> Product4/1
  Rotor State1/1 -> Switch/3
  Step/1 -> Switch/2
  Rotor_Speed_Vector/1 -> Product4/2
  Product2/1 -> Thrust_N_Moment/1
  Sum_Rotor_Angular_Velocity_Mat1/1 -> Product3/1
  Product3/1 -> Sum of Elements/1
  Sum of Elements/1 -> Omega/1

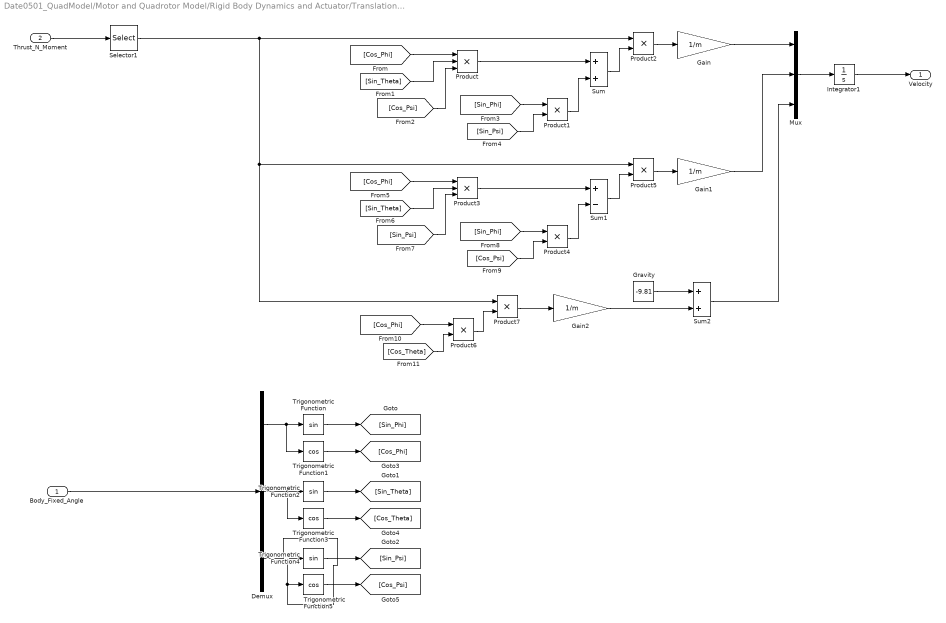
== system Date0501_QuadModel/Motor and Quadrotor Model/Rigid Body Dynamics and Actuator/Translation Dynamic ==
  Body_Fixed_Angle : Inport
  Thrust_N_Moment : Inport  Port=2
  Demux : Demux  Outputs=3
  Gain : Gain  Gain=1/m
  Gain1 : Gain  Gain=1/m
  Gain2 : Gain  Gain=1/m
  Gravity : Constant  Value=-9.81
  Integrator1 : Integrator  InitialCondition=[0 0 0]
  Mux : Mux  Inputs=3
  Product : Product  Inputs=3
  Product{1..2,4..7} (6 alike) : Product
  Product3 : Product  Inputs=3
  Selector1 : Selector  InputPortWidth=4  Indices=[1]
  Sum : Sum
  Sum1 : Sum  Inputs=+-
  Sum2 : Sum
  Trigonometric Function : Trigonometry
  Trigonometric Function1 : Trigonometry  Operator=cos
  Trigonometric Function2 : Trigonometry
  Trigonometric Function3 : Trigonometry  Operator=cos
  Trigonometric Function4 : Trigonometry
  Trigonometric Function5 : Trigonometry  Operator=cos
  Velocity : Outport
  wires:
  Body_Fixed_Angle/1 -> Demux/1
  Demux/1 -> Trigonometric Function/1, Trigonometric Function1/1
  Trigonometric Function/1 -> [Sin_Phi]
  Trigonometric Function1/1 -> [Cos_Phi]
  Demux/2 -> Trigonometric Function3/1, Trigonometric Function2/1
  Trigonometric Function2/1 -> [Sin_Theta]
  Trigonometric Function3/1 -> [Cos_Theta]
  Trigonometric Function4/1 -> [Sin_Psi]
  Trigonometric Function5/1 -> [Cos_Psi]
  Demux/3 -> Trigonometric Function4/1, Trigonometric Function5/1
  [Cos_Phi] -> Product/1
  [Sin_Theta] -> Product/2
  [Cos_Psi] -> Product/3
  Product/1 -> Sum/1
  [Sin_Phi] -> Product1/1
  [Sin_Psi] -> Product1/2
  Product1/1 -> Sum/2
  Sum/1 -> Product2/2
  Product2/1 -> Gain/1
  [Cos_Phi] -> Product3/1
  [Sin_Theta] -> Product3/2
  [Sin_Psi] -> Product3/3
  Product3/1 -> Sum1/1
  [Sin_Phi] -> Product4/1
  [Cos_Psi] -> Product4/2
  Product4/1 -> Sum1/2
  Sum1/1 -> Product5/2
  Selector1/1 -> Product7/1, Product5/1, Product2/1
  Product5/1 -> Gain1/1
  Gain1/1 -> Mux/2
  [Cos_Phi] -> Product6/1
  [Cos_Theta] -> Product6/2
  Product7/1 -> Gain2/1
  Gain2/1 -> Sum2/2
  Gravity/1 -> Sum2/1
  Product6/1 -> Product7/2
  Gain/1 -> Mux/1
  Sum2/1 -> Mux/3
  Mux/1 -> Integrator1/1
  Integrator1/1 -> Velocity/1
  Thrust_N_Moment/1 -> Selector1/1
